simulink model "fonctionnel"  (R2024a)
settings: Solver=ode23t  StartTime=0.0  StopTime=24  RelTol=1e-3
PreLoadFcn:
  | addpath('Resources')
undefined symbols (not defined in the file or in its folder): DiscIntNeverNeededParam
libraries: simulink x6, spsThreePhaseDynamicLoadLib x3, spsThreePhaseVIMeasurementLib x3, spsThreePhaseBreakerLib x3, spsPower3phPhasorLib x2, spsThreePhaseSourceLib x2, SignalEditorBlockLib x1, spsThreePhaseSeriesRLCLoadLib x1, spsThreePhaseTransformerTwoWindingsLib x1, sps_lib x1, powerlib_meascontrol x1, powerlib x1
(part 2 of 2)

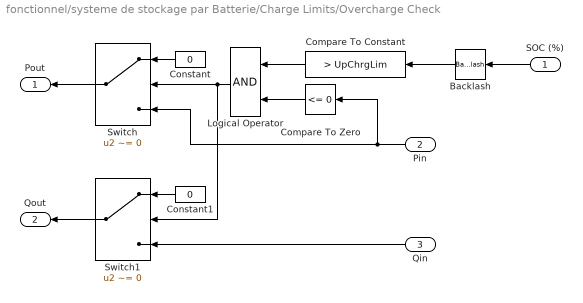
== system fonctionnel/systeme de stockage par Batterie/Charge Limits/Overcharge Check ==
  SOC (%) : Inport
  Pin : Inport  Port=2
  Qin : Inport  Port=3
  Backlash : Backlash  BacklashWidth=1e-3  InitialOutput=Initial_kWh_pc  ZeroCross=off
  Compare To Constant : simulink/Logic and Bit Operations/Compare To Constant  relop=>  const=UpChrgLim  OutDataTypeStr=boolean
  Compare To Zero : simulink/Logic and Bit Operations/Compare To Zero  relop=<=  OutDataTypeStr=boolean
  Constant : Constant  Value=0
  Constant1 : Constant  Value=0
  Logical Operator : Logic  AllPortsSameDT=off  OutDataTypeStr=boolean
  Switch : Switch  Criteria=u2 ~= 0  SaturateOnIntegerOverflow=off  InputSameDT=off
  Switch1 : Switch  Criteria=u2 ~= 0  SaturateOnIntegerOverflow=off  InputSameDT=off
  Pout : Outport  VectorParamsAs1DForOutWhenUnconnected=off
  Qout : Outport  Port=2  VectorParamsAs1DForOutWhenUnconnected=off
  wires:
  Backlash/1 -> Compare To Constant/1
  Switch1/1 -> Qout/1
  Constant1/1 -> Switch1/1
  Qin/1 -> Switch1/3
  Compare To Zero/1 -> Logical Operator/2
  Switch/1 -> Pout/1
  Pin/1 -> Switch/3, Compare To Zero/1
  SOC (%)/1 -> Backlash/1
  Constant/1 -> Switch/1
  Logical Operator/1 -> Switch/2, Switch1/2
  Compare To Constant/1 -> Logical Operator/1

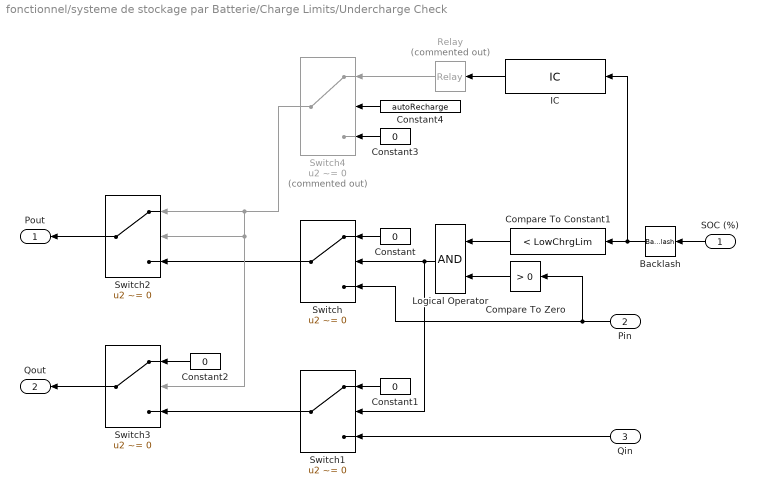
== system fonctionnel/systeme de stockage par Batterie/Charge Limits/Undercharge Check ==
  SOC (%) : Inport
  Pin : Inport  Port=2
  Qin : Inport  Port=3
  Backlash : Backlash  BacklashWidth=1e-3  InitialOutput=Initial_kWh_pc  ZeroCross=off
  Compare To Constant1 : simulink/Logic and Bit Operations/Compare To Constant  relop=<  const=LowChrgLim  OutDataTypeStr=boolean
  Compare To Zero : simulink/Logic and Bit Operations/Compare To Zero  relop=>  OutDataTypeStr=boolean
  Constant{,1..3} (4 alike) : Constant  Value=0
  Constant4 : Constant  Value=autoRecharge
  IC : InitialCondition  Value=RechargeSOC
  Logical Operator : Logic  AllPortsSameDT=off  OutDataTypeStr=boolean
  Relay : Relay  Commented=on  OnSwitchValue=RechargeSOC  OffSwitchValue=LowChrgLim  OnOutputValue=0  OffOutputValue=-Precharge/100*Pnom
  Switch{,1..3} (4 alike) : Switch  Criteria=u2 ~= 0  SaturateOnIntegerOverflow=off  InputSameDT=off
  Switch4 : Switch  Commented=on  Criteria=u2 ~= 0  SaturateOnIntegerOverflow=off  InputSameDT=off
  Pout : Outport  VectorParamsAs1DForOutWhenUnconnected=off
  Qout : Outport  Port=2  VectorParamsAs1DForOutWhenUnconnected=off
  wires:
  Constant4/1 -> Switch4/2
  Constant3/1 -> Switch4/3
  Relay/1 -> Switch4/1
  Constant2/1 -> Switch3/1
  Switch1/1 -> Switch3/3
  Switch3/1 -> Qout/1
  Switch2/1 -> Pout/1
  Switch/1 -> Switch2/3
  IC/1 -> Relay/1
  Switch4/1 -> Switch3/2, Switch2/2, Switch2/1
  Backlash/1 -> Compare To Constant1/1, IC/1
  Qin/1 -> Switch1/3
  Constant1/1 -> Switch1/1
  Compare To Constant1/1 -> Logical Operator/1
  Logical Operator/1 -> Switch1/2, Switch/2
  Constant/1 -> Switch/1
  SOC (%)/1 -> Backlash/1
  Pin/1 -> Compare To Zero/1, Switch/3
  Compare To Zero/1 -> Logical Operator/2

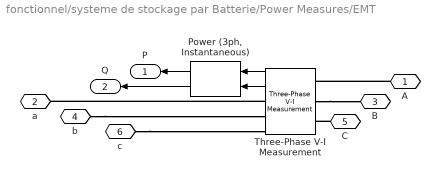
== system fonctionnel/systeme de stockage par Batterie/Power Measures/EMT ==
  "Power (3ph, Instantaneous)" : powerlib_meascontrol/Measurements/Power (3ph, Instantaneous)
      settings: SourceProductName=Simscape Electrical
  Three-Phase V-I Measurement : powerlib/Measurements/Three-Phase V-I Measurement  VoltageMeasurement=phase-to-ground  SetLabelV=off  LabelV=Vabc  Vpu=off  VpuLL=off  CurrentMeasurement=yes  SetLabelI=off  LabelI=Iabc  Ipu=off  Pbase=100e6  Vbase=500e3  OutputType=Complex  PhasorSimulation=on  PSBequivalent=0
      settings: SourceProductName=Simscape Electrical
  A : PMIOPort  Side=Left
  a : PMIOPort  Port=2  Side=Right
  B : PMIOPort  Port=3  Side=Left
  b : PMIOPort  Port=4  Side=Right
  C : PMIOPort  Port=5  Side=Left
  c : PMIOPort  Port=6  Side=Right
  P : Outport  VectorParamsAs1DForOutWhenUnconnected=off
  Q : Outport  Port=2  VectorParamsAs1DForOutWhenUnconnected=off
  wires:
  Three-Phase V-I Measurement/2 -> "Power (3ph, Instantaneous)"/2
  Three-Phase V-I Measurement/1 -> "Power (3ph, Instantaneous)"/1
  "Power (3ph, Instantaneous)"/1 -> P/1
  "Power (3ph, Instantaneous)"/2 -> Q/1
  connections:
  Three-Phase V-I Measurement/RConn1 -- a/RConn1
  b/RConn1 -- Three-Phase V-I Measurement/RConn2
  A/RConn1 -- Three-Phase V-I Measurement/LConn1
  Three-Phase V-I Measurement/LConn2 -- B/RConn1
  c/RConn1 -- Three-Phase V-I Measurement/RConn3
  C/RConn1 -- Three-Phase V-I Measurement/LConn3

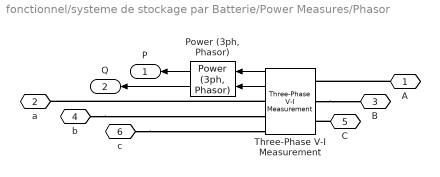
== system fonctionnel/systeme de stockage par Batterie/Power Measures/Phasor ==
  "Power (3ph, Phasor)" : spsPower3phPhasorLib/Power (3ph, Phasor)
      settings: LibrarySourceBlock=|
      | sps_lib/Sensors and Measurements/Power
      | (3ph, Phasor)
  Three-Phase V-I Measurement : spsThreePhaseVIMeasurementLib/Three-Phase V-I Measurement  VoltageMeasurement=phase-to-ground  SetLabelV=off  LabelV=Vabc  Vpu=off  VpuLL=off  CurrentMeasurement=yes  SetLabelI=off  LabelI=Iabc  Ipu=off  Pbase=100e6  Vbase=500e3  OutputType=Complex  PhasorSimulation=on  PSBequivalent=0
  A : PMIOPort  Side=Left
  a : PMIOPort  Port=2  Side=Right
  B : PMIOPort  Port=3  Side=Left
  b : PMIOPort  Port=4  Side=Right
  C : PMIOPort  Port=5  Side=Left
  c : PMIOPort  Port=6  Side=Right
  P : Outport  VectorParamsAs1DForOutWhenUnconnected=off
  Q : Outport  Port=2  VectorParamsAs1DForOutWhenUnconnected=off
  wires:
  "Power (3ph, Phasor)"/2 -> Q/1
  "Power (3ph, Phasor)"/1 -> P/1
  Three-Phase V-I Measurement/1 -> "Power (3ph, Phasor)"/1
  Three-Phase V-I Measurement/2 -> "Power (3ph, Phasor)"/2
  connections:
  C/RConn1 -- Three-Phase V-I Measurement/LConn3
  c/RConn1 -- Three-Phase V-I Measurement/RConn3
  Three-Phase V-I Measurement/LConn2 -- B/RConn1
  A/RConn1 -- Three-Phase V-I Measurement/LConn1
  b/RConn1 -- Three-Phase V-I Measurement/RConn2
  Three-Phase V-I Measurement/RConn1 -- a/RConn1

== stateflow chart fonctionnel/EMS/Chart ==
  state Systeme_de_gestion_d_energie
    during : P_net = P_pv - P_load; % Puissance nette (pour transitions)
    state ACHAT_RESEAU
      entry : P_bat_ref = 0; mode = 4; P_grid = 0;
      during : P_pv_ref = min(P_pv, P_load); % 1) Puissance PV utilisée pour la charge
      P_deficit = P_load - P_pv_ref; % 2) Déficit de puissance
      % 3) Gestion batterie
      if SOC < SOC_min
      % Batterie protégée → recharge obligatoire
      P_bat_ref = P_ch_max;     % charge batterie (positive)
      elseif SOC < SOC_max
      % Batterie normale → recharge possible
      P_bat_ref = min(P_ch_max, P_grid_max);
      else
      % Batterie pleine
      P_bat_ref = 0;
      end
      % 4) Puissance réseau = charge + recharge batterie
      P_grid = P_deficit + P_bat_ref;
    state CHARGE_ET_VENTE_RESEAU
      entry: mode = 6;
      P_grid = 0;
      P_bat_ref = 0;
      during : % PV alimente la charge en priorité
      P_pv_ref = min(P_pv, P_load);
      % surplus PV
      P_surplus = P_pv - P_pv_ref;
      % 1) Charge batterie si possible
      if SOC < SOC_max
      P_bat_ref = min(P_surplus, P_ch_max);    % positif = charge
      else
      P_bat_ref = 0;
      end
      % 2) Vendre le surplus restant au réseau (si réseau disponible)
      if grid_on == 1
      P_restant = P_surplus - P_bat_ref;       % ce qui reste après charge batt
      if P_restant > 0
      P_grid = -P_restant;                 % négatif = vente (export)
      else
      P_grid = 0;
      end
      else
      P_grid = 0;   % réseau coupé => pas de vente
      end
    state PV_ALIMENTE_CHARGE
      entry:
      P_bat_ref = 0;
      P_grid = 0;
      during : mode =1;
      P_pv_ref = min(P_pv, P_load);
    state CHARGE_BATTERIE_vente_surplus
      entry:
      P_grid = 0;
      during: mode =2;
      P_pv_ref = min(P_pv, P_load);
      P_surplus = P_pv - P_pv_ref;
      P_bat_ref = min(P_surplus, P_ch_max);
      P_grid =  -(P_pv-P_pv_ref-P_bat_ref);
    state DECHARGE_BATTERIE
      entry:
      P_grid = 0;
      P_bat_ref = 0;
      during: mode = 3;
      % 1) Puissance PV réellement utilisée
      P_pv_ref = min(P_pv, P_load);
      % 2) Déficit de puissance
      P_deficit = P_load - P_pv_ref;
      % 3) Protection SOC : ne pas décharger si batterie trop basse
      if SOC <= SOC_min
      P_bat_ref = 0;
      else
      % Décharge batterie (puissance négative)
      P_bat_ref = -min(P_deficit, P_dis_max);
      end
      % 4) Gestion du réseau
      if grid_on == 1
      % Le réseau fournit ce que la batterie ne peut pas fournir
      P_grid = P_deficit - (-P_bat_ref);
      else
      % Réseau coupé
      P_grid = 0;
      end
    state VENTE_SEULE
      entry: mode = 7;
      P_bat_ref = 0;
      P_grid = 0;
      during: P_pv_ref = min(P_pv, P_load);
      P_surplus = P_pv - P_pv_ref;
      % Batterie pleine => pas de charge
      P_bat_ref = 0;
      % Vendre tout le surplus
      if grid_on == 1 && P_surplus > 0
      P_grid = -P_surplus;
      else
      P_grid = 0;
      end
    state MODE_ILOTAGE
      entry : P_grid = 0; mode = 5;
      during : P_pv_ref = min(P_pv, P_load);
      P_deficit = P_load - P_pv_ref;
      if SOC > SOC_min
      P_bat_ref = -min(P_deficit, P_dis_max);
      P_non_alimente = max(0, P_deficit - (-P_bat_ref));
      else
      P_bat_ref = 0;
      P_non_alimente = P_deficit;
      P_grid = P_non_alimente;
      P_net = P_pv - P_load;
      end
    note: Convention des puissances (signes)
    note: P_pv​≥0 : puissance PV disponible
        | P_pv_ref≥0 : puissance PV réellement utilisée
        | (vers charge + éventuellement batterie)
    note: Pgrid​>0 : achat / import depuis le réseau
        | Pgrid<0 : vente / export vers le réseau
        | Pgrid=0 : réseau non utilisé / coupé
    note: P_bat_ref​>0 : charge de la batterie
        | P_bat_ref<0 : décharge de la batterie
        | P_bat_ref=0 : batterie neutre
    (default) -> PV_ALIMENTE_CHARGE
    ACHAT_RESEAU -> DECHARGE_BATTERIE [order 3] : [SOC > SOC_min + 2 && P_net < -epsP]
    ACHAT_RESEAU -> PV_ALIMENTE_CHARGE [order 1] : [P_net >= -epsP]
    PV_ALIMENTE_CHARGE -> ACHAT_RESEAU [order 4] : [P_net < -epsP && SOC <= SOC_min]
    ACHAT_RESEAU -> MODE_ILOTAGE [order 4] : [grid_on == 0]
    CHARGE_BATTERIE_vente_surplus -> ACHAT_RESEAU [order 3] : [P_net < -epsP && SOC <= SOC_min]
    ACHAT_RESEAU -> CHARGE_BATTERIE_vente_surplus [order 2] : [P_net > epsP && SOC < SOC_max]
    CHARGE_BATTERIE_vente_surplus -> CHARGE_ET_VENTE_RESEAU [order 4] : [grid_on==1 && (P_pv - min(P_pv,P_load)) > P_ch_max && SOC < SOC_max]
    PV_ALIMENTE_CHARGE -> CHARGE_BATTERIE_vente_surplus [order 1] : [P_net > epsP && SOC < SOC_max]
    CHARGE_BATTERIE_vente_surplus -> PV_ALIMENTE_CHARGE [order 1] : [P_net <= epsP || SOC >= SOC_max]
    CHARGE_ET_VENTE_RESEAU -> CHARGE_BATTERIE_vente_surplus [order 1] : [(P_pv - min(P_pv,P_load)) <= P_ch_max || grid_on==0]
    CHARGE_BATTERIE_vente_surplus -> DECHARGE_BATTERIE [order 2] : [P_net < -epsP && SOC > SOC_min]
    MODE_ILOTAGE -> CHARGE_BATTERIE_vente_surplus [order 1] : [grid_on == 1 && P_net > epsP && SOC < SOC_max]
    CHARGE_ET_VENTE_RESEAU -> PV_ALIMENTE_CHARGE [order 2] : [P_net <= epsP]
    PV_ALIMENTE_CHARGE -> CHARGE_ET_VENTE_RESEAU [order 5] : [grid_on==1 && P_net > epsP && SOC < SOC_max]
    DECHARGE_BATTERIE -> PV_ALIMENTE_CHARGE [order 1] : [P_net >= -epsP]
    PV_ALIMENTE_CHARGE -> DECHARGE_BATTERIE [order 3] : [P_net < -epsP && SOC > SOC_min]
    MODE_ILOTAGE -> PV_ALIMENTE_CHARGE [order 3] : [grid_on == 1]
    PV_ALIMENTE_CHARGE -> MODE_ILOTAGE [order 2] : [grid_on == 0]
    VENTE_SEULE -> PV_ALIMENTE_CHARGE [order 1] : [P_net <= epsP]
    PV_ALIMENTE_CHARGE -> VENTE_SEULE [order 6] : [grid_on==1 && P_net > epsP && SOC >= SOC_max]
    VENTE_SEULE -> CHARGE_ET_VENTE_RESEAU [order 2] : [SOC < SOC_max && P_net > epsP && grid_on==1]
    CHARGE_ET_VENTE_RESEAU -> VENTE_SEULE [order 3] : [SOC >= SOC_max && P_net > epsP && grid_on==1]
    MODE_ILOTAGE -> DECHARGE_BATTERIE [order 2] : [grid_on == 1 && P_net < -epsP && SOC > SOC_min]
    DECHARGE_BATTERIE -> MODE_ILOTAGE [order 2] : [SOC <= SOC_min && ~grid_on]
  (default) -> Systeme_de_gestion_d_energie : {P_net = P_pv - P_load;} % Puissance nette (pour transitions)
  data: P_pv input; P_load input; P_pv_ref output; P_bat_ref output; P_grid output; P_net output; P_ch_max local =5; P_surplus local; epsP constant double =0.2; SOC input; SOC_max constant double =90; mode output; grid_on input; P_dis_max local =5; P_deficit local; SOC_min constant double =10; P_non_alimente output; P_restant output; P_grid_max constant double =12

== matlab function fonctionnel/EMS/MATLAB Function ==
  data: mode input; modeText output
function modeText = mode_to_text(mode)
% mode : entier venant de l'EMS

% Initialisation obligatoire (sécurité Simulink)
modeText = "Inconnu";

switch mode
    case 1
        modeText = "PV alimente charge";
    case 2
        modeText = "Charge batterie";
    case 3
        modeText = "Decharge batterie";
    case 4
        modeText = "Achat reseau";
    case 5
        modeText = "Mode Ilote";
    case 6
        modeText = "Vente reseau";
    otherwise
        modeText = "Mode non defini";
end
